simulink model "Granulometria_bloqueh5"  (R2015a)
settings: Solver=ode45  StartTime=0.0  StopTime=50  RelTol=1e-3
settings Model: Creator=Fer  LastModifiedBy=Fer

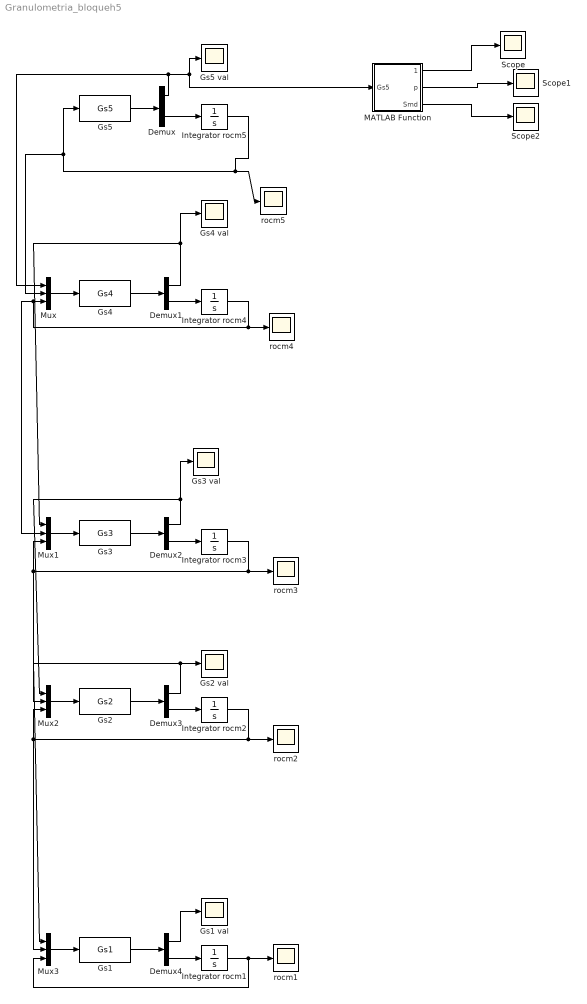
== system Granulometria_bloqueh5 ==
  Demux{,1..4} (5 alike) : Demux  Outputs=2
  Gs1 : MATLABFcn  MATLABFcn=Gs1
  Gs1 val : Scope
      settings: SaveName=ScopeData8
  Gs2 : MATLABFcn  MATLABFcn=Gs2
  Gs2 val : Scope
      settings: SaveName=ScopeData6
  Gs3 : MATLABFcn  MATLABFcn=Gs3
  Gs3 val : Scope
      settings: SaveName=ScopeData4
  Gs4 : MATLABFcn  MATLABFcn=Gs4
  Gs4 val : Scope
      settings: SaveName=ScopeData2
  Gs5 : MATLABFcn  MATLABFcn=Gs5
  Gs5 val : Scope
  Integrator rocm{1..5} (5 alike) : Integrator  InitialCondition=1.6
  MATLAB Function : MATLAB Function  TreatAsAtomicUnit=on
  Mux{,1..3} (4 alike) : Mux  Inputs=3
  Scope : Scope
      settings: SaveName=ScopeData10
  Scope1 : Scope
      settings: SaveName=ScopeData11
  Scope2 : Scope
      settings: SaveName=ScopeData12
  rocm{1..5} (5 alike) : Scope
      rocm1 settings: SaveName=ScopeData9
      rocm2 settings: SaveName=ScopeData7
      rocm3 settings: SaveName=ScopeData5
      rocm4 settings: SaveName=ScopeData3
  wires:
  Integrator rocm5/1 -> rocm5/1, Gs5/1, Mux/2
  Gs5/1 -> Demux/1
  Demux/2 -> Integrator rocm5/1
  Demux/1 -> Mux/1, MATLAB Function/1(Gs5), Gs5 val/1
  Gs4/1 -> Demux1/1
  Demux1/2 -> Integrator rocm4/1
  Demux1/1 -> Gs4 val/1, Mux1/1
  Integrator rocm4/1 -> rocm4/1, Mux1/2, Mux/3
  Mux/1 -> Gs4/1
  Gs3/1 -> Demux2/1
  Demux2/2 -> Integrator rocm3/1
  Mux1/1 -> Gs3/1
  Demux2/1 -> Gs3 val/1, Mux2/1
  Integrator rocm3/1 -> rocm3/1, Mux1/3, Mux2/2
  Mux2/1 -> Gs2/1
  Gs2/1 -> Demux3/1
  Demux3/1 -> Gs2 val/1, Mux3/1
  Demux3/2 -> Integrator rocm2/1
  Integrator rocm2/1 -> rocm2/1, Mux2/3, Mux3/2
  Mux3/1 -> Gs1/1
  Gs1/1 -> Demux4/1
  Demux4/2 -> Integrator rocm1/1
  Demux4/1 -> Gs1 val/1
  Integrator rocm1/1 -> Mux3/3, rocm1/1
  MATLAB Function/1(fptHPGRu) -> Scope/1
  MATLAB Function/2(p) -> Scope1/1
  MATLAB Function/3(Smd) -> Scope2/1

== matlab function Granulometria_bloqueh5/MATLAB Function ==
  data: Gs5 input; fptHPGRu output; p output; Smd output
function [fptHPGRu,p,Smd] = Granulometria_bloqueh5(Gs5) 
% #codegen
n=0;
U=0;
NB=0;
Ppb=0;
h=0;
SiE=[0];
fipHPGR=[0];
b=[0];
A=[0];
S=[0];
p=[0];
fptHPGR=[0];
fpeHPGR=[0];
fpcHPGR=[0];
fptHPGRu=[0];
fpeHPGRu=[0];
fpcHPGRu=[0];
coder.extrinsic('evalin');
U=evalin('base','U');
n=evalin('base','n');
NB=evalin('base','NB');
Ppb=evalin('base','Ppb');
b=evalin('base','b');
SiE=evalin('base','SiE');
fipHPGR=evalin('base','fipHPGR');
h=evalin('base','h');
Hkb1 = (1/NB)*Gs5*h/(3600*U);
%velocidad específica de fractura para cada tamaño en cada bloque: S(i,k)
for i = 1:n;
    for k = 1:NB;
        S(i,k) = (Ppb(k)/Hkb1)*SiE(i)/3600; %S(i,k) en [1/s]
    end
end
%Variables de entrada para modelar la Matriz de REID:
%Valores de partida
A(1,1) = fipHPGR(1);
%MATRIZ DE REID CONDICIONES
for i=1:n,
    for j=1:n,
        if i<j,
            A(i,j) = 0;
        else if i>j,
                suma = 0;
                for l=j:i-1,
                    suma = suma + b(i,l)*SiE(l)*A(l,j)/(SiE(i)-SiE(j));
                    A(i,j) = suma;
                end
            else i=j;
                suma = 0;
                for l=1:i-1,
                    suma = suma + A(i,l);
                    A(i,j) = fipHPGR(i) - suma;
                end
            end
        end
    end
end
%Distribución del tamaño de partícula en zona BP,
%Granulometria por bloques 
for k = 1:NB;
    for i = 1:n-1;
        suma = 0;
        for j = 1:i;
            suma = suma + A(i,j)*exp(-1*S(j,k)*h/U);% Distribución granulométrica ec 3.29
            %de producto de la zona de compresión de capas de partículas, para cada bloque k, [ton(i)/ton
            p(i,k) = suma;
        end
    end
    for i = n;
        p(i,k) = 1 - sum(p(1:n-1,k));
    end
end
%Distribucion de tamaño de partícula total HPGR: f(i)ptHPGR en [ton(i)/tonT]
for i = 1:n;
    suma = 0;
    for k = 1:NB;
        suma = suma + p(i,k); %Sumatoria de las fracciones másicas divididas para el NB
        fptHPGR(i) = suma/NB; %GRANULOMETRIA DE PRODUCTO TOTAL DEL HPGR
    end
end
%Distribución de tamaño de partícula bordes del HPGR: f(i)peHPGR en
%[ton(i)/tonT]
a = 0.24; %Parámetro fracción en peso que circula en los bordes
E = 0.5*a*NB; %N° de bloques, E, correspondiente a los bordes
for i=1:n;
    suma = 0;
    for k = 1:round(E);
        suma = suma + p(i,k);
    end
    fpeHPGR(i) = (suma + (E - round(E))*p(i,round(E)+1))/E;
    %GRANULOMETRIA DE PRODUCTO CHANCADO POR EFECTO DE BORDE
end
%Distribución de tamaño de partícula centro del HPGR: f(i)pcHPGR en
%[ton(i)/tonT]
for i = 1:n;
    fpcHPGR(i) = (fptHPGR(i) - a*fpeHPGR(i))/(1-a);
    %GRANULOMETRIA DE PRODUCTO CHANCADO POR COMPRESION DE CAPAS DE
    %PARTICULAS
end
%Distribución de tamaño de productos en forma acumulada pasante
for i = 1;
    fptHPGRu(i) = 1;
    fpeHPGRu(i) = 1;
    fpcHPGRu(i) = 1;
end
for i = 2:n;
    fptHPGRu(i) = fptHPGRu(i-1) - fptHPGR(i-1);
    fpeHPGRu(i) = fpeHPGRu(i-1) - fpeHPGR(i-1);
    fpcHPGRu(i) = fpcHPGRu(i-1) - fpcHPGR(i-1);
end
fptHPGRu(1:n) = fptHPGRu(1:n)*100;
fpeHPGRu(1:n) = fpeHPGRu(1:n)*100;
fpcHPGRu(1:n) = fpcHPGRu(1:n)*100;
%Conversion de S a [1/h]
Smd = S*3600;
end
